simulink model "gemini_davide_sim"  (R2025b)
settings: Solver=VariableStepAuto  StartTime=0.0  StopTime=t_sim  RelTol=1e-3
values from neighbouring files (symbols this model uses):
  delta_d1 = 0    [gemini_davide.m]
  delta_d2 = 4    [gemini_davide.m]
  delta_r = 0    [gemini_davide.m]
  Ts = 0.05    [gemini_davide.m]
undefined symbols (not defined in the file or in its folder): DiscIntNeverNeededParam
libraries: cstblocks x2
settings Model: Creator=giovannimasi  LastModifiedBy=giovannimasi

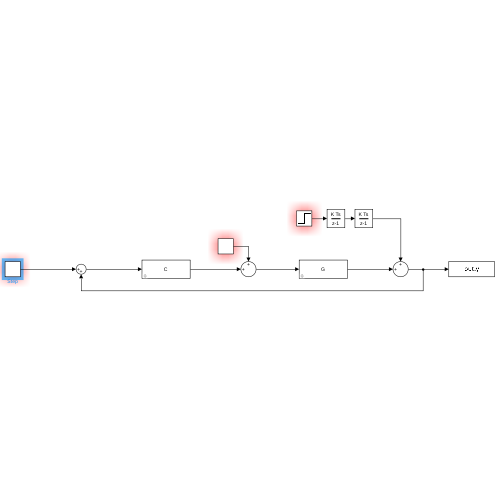
[thumbnail: Simulink's stored preview of the top-level diagram]
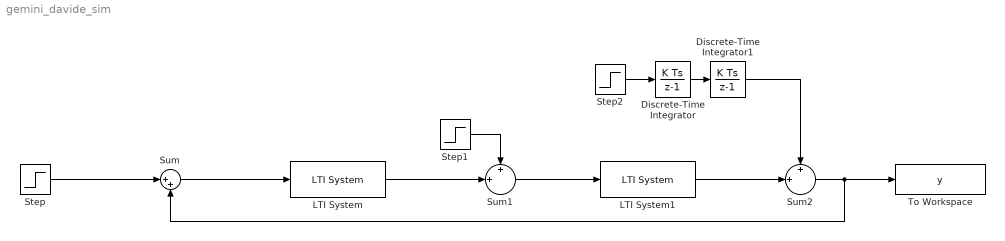
== system gemini_davide_sim ==
  Discrete-Time Integrator : DiscreteIntegrator  SampleTime=-1  ICPrevOutput=DiscIntNeverNeededParam  ICPrevScaledInput=DiscIntNeverNeededParam
  Discrete-Time Integrator1 : DiscreteIntegrator  SampleTime=-1  ICPrevOutput=DiscIntNeverNeededParam  ICPrevScaledInput=DiscIntNeverNeededParam
  LTI System : cstblocks/LTI System  sys=C  IC=[]  PadeOrder=0
  LTI System1 : cstblocks/LTI System  sys=G  IC=[]  PadeOrder=0
  Step : Step  Time=0  After=delta_r  SampleTime=Ts
  Step1 : Step  Time=0  After=delta_d1  SampleTime=Ts
  Step2 : Step  Time=0  After=delta_d2  SampleTime=Ts
  Sum : Sum  Inputs=|++
  Sum1 : Sum  Inputs=+|+||
  Sum2 : Sum  Inputs=+|+||
  To Workspace : ToWorkspace  VariableName=y  SaveFormat=Timeseries  SampleTime=Ts
  wires:
  Step/1 -> Sum/1
  Sum/1 -> LTI System/1
  LTI System/1 -> Sum1/2
  Sum1/1 -> LTI System1/1
  LTI System1/1 -> Sum2/2
  Sum2/1 -> Sum/2, To Workspace/1
  Step1/1 -> Sum1/1
  Step2/1 -> Discrete-Time Integrator/1
  Discrete-Time Integrator/1 -> Discrete-Time Integrator1/1
  Discrete-Time Integrator1/1 -> Sum2/1
